simulink model "seminar5_topic1"  (R2019b)
settings: Solver=VariableStepAuto  StartTime=0.0  StopTime=0.08  RelTol=1e-3
libraries: powerlib x9, powerlib_meascontrol x1
settings Model: Creator=96547  LastModifiedBy=96547
settings DataIOCC: ReturnWorkspaceOutputs=off

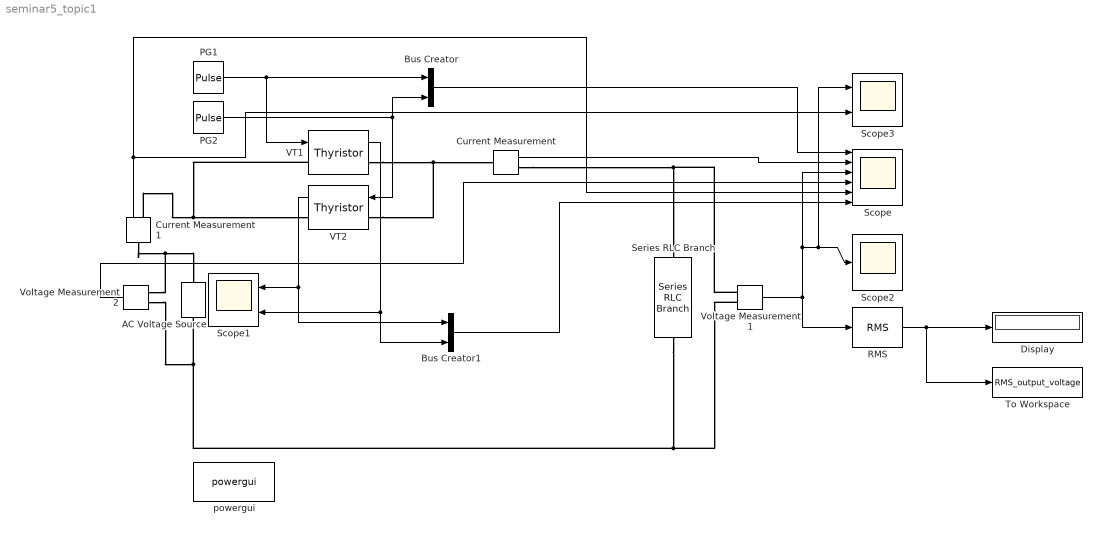
== system seminar5_topic1 ==
  AC Voltage Source : powerlib/Electrical Sources/AC Voltage Source  Amplitude=220*sqrt(2)  Phase=0  Frequency=50  SampleTime=0  Measurements=None  BusType=swing  Pref=10e3  Qref=0  Qmin=-inf  Qmax=+inf
      settings: SourceProductName=Simscape Electrical
  Bus Creator : BusCreator  Inputs=2
  Bus Creator1 : BusCreator  Inputs=2
  Current Measurement : powerlib/Measurements/Current Measurement  PhasorSimulation=off  OutputType=Complex  PSBequivalent=0
      settings: SourceProductName=Simscape Electrical
  Current Measurement1 : powerlib/Measurements/Current Measurement  PhasorSimulation=off  OutputType=Complex  PSBequivalent=0
      settings: SourceProductName=Simscape Electrical
  Display : Display
  PG1 : DiscretePulseGenerator  PulseType=Time based  Period=0.02  PulseWidth=50  PhaseDelay=(90/360)*0.02
  PG2 : DiscretePulseGenerator  PulseType=Time based  Period=0.02  PulseWidth=50  PhaseDelay=(90/360)*0.02+0.01
  RMS : powerlib_meascontrol/Measurements/RMS  TrueRMS=on  Freq=50  RMSInit=120  Ts=0
      settings: SourceProductName=Simscape Electrical
  Scope : Scope  NumInputPorts=6
  Scope1 : Scope  NumInputPorts=2
  Scope2 : Scope
  Scope3 : Scope  NumInputPorts=2
  Series RLC Branch : powerlib/Elements/Series RLC Branch  LConnTagsString=__new0  RConnTagsString=__new0  BranchType=RL  Resistance=10  Inductance=2.2e-3  SetiL0=off  InitialCurrent=0  Capacitance=1e-6  Setx0=off  InitialVoltage=0  Measurements=None
      settings: SourceProductName=Simscape Electrical
  To Workspace : ToWorkspace  VariableName=RMS_output_voltage  SampleTime=-1
      settings: Save2DSignal=2-D array (concatenate along first dimension)
  VT1 : powerlib/Power Electronics/Thyristor  Ron=0  Lon=0  Vf=0.8  IC=0  Rs=500  Cs=250e-9  Measurements=on
      settings: SourceProductName=Simscape Electrical
  VT2 : powerlib/Power Electronics/Thyristor  Ron=0  Lon=0  Vf=0.8  IC=0  Rs=500  Cs=250e-9  Measurements=on
      settings: SourceProductName=Simscape Electrical
  Voltage Measurement1 : powerlib/Measurements/Voltage Measurement  PhasorSimulation=off  OutputType=Complex  PSBequivalent=0
      settings: SourceProductName=Simscape Electrical
  Voltage Measurement2 : powerlib/Measurements/Voltage Measurement  PhasorSimulation=off  OutputType=Complex  PSBequivalent=0
      settings: SourceProductName=Simscape Electrical
  powergui : powerlib/powergui  Priority=1  SimulationMode=Continuous  SampleTime=50e-6  frequency=60  Iterations=50  frequencyindice=50  Pbase=100e6  ErrMax=1e-4  UnitsV=kV  UnitsW=MW  buscounter=0  FunctionMessages=off  echomessages=off  EnableUseOfTLC=off  CurrentSourceSwitches=off  DisableSnubberDevices=off  DisableRonSwitches=off  DisableVfSwitches=off  DisplayEquations=off  AutomaticDiscreteSolvers=off  SolverType=Tustin/Backward Euler (TBE)  Interpol=off  ExternalGateDelay=off  methode=off  Ts=100  x0status=blocks  SPID=on  SwTol=0  HookPort=off  NonlinearTolerance=1e-4  nMaxIteration=100  ContinueOnMaxIteration=off  RestoreLinks=warning  ResistiveCurrentMeasurement=off  Frange=[0:2:500]  Ylog=off  Xlog=on  ShowGrid=off  save=off  variable=ZData  structure=output_voltage  ZoomFFT=on  StartTime=0.0  cycles=4  DisplayStyle=1  fundamental=50  FreqAxis=on  MaxFrequency=500  frequencyindicesteady=1  RmsSteady=1  display=off
      settings: SourceProductName=Simscape Electrical
  wires:
  PG1/1 -> Bus Creator/1, VT1/1
  PG2/1 -> VT2/1, Bus Creator/2
  RMS/1 -> To Workspace/1, Display/1
  Voltage Measurement1/1 -> Scope3/1, Scope2/1, Scope/3, RMS/1
  Current Measurement/1 -> Scope/2
  VT2/1 -> Bus Creator1/1, Scope1/1
  VT1/1 -> Bus Creator1/2, Scope1/2
  Bus Creator/1 -> Scope/1
  Voltage Measurement2/1 -> Scope/4
  Current Measurement1/1 -> Scope3/2, Scope/5
  Bus Creator1/1 -> Scope/6
  connections:
  VT1/RConn1 -- VT2/LConn1 -- Current Measurement/LConn1
  Current Measurement/RConn1 -- Series RLC Branch/LConn1 -- Voltage Measurement1/LConn1
  Series RLC Branch/RConn1 -- Voltage Measurement1/LConn2 -- Voltage Measurement2/LConn1 -- AC Voltage Source/LConn1
  Voltage Measurement2/LConn2 -- AC Voltage Source/RConn1 -- Current Measurement1/LConn1
  VT1/LConn1 -- VT2/RConn1 -- Current Measurement1/RConn1
